simulink model "archSystemMQTT"  (R2021b)
settings: Solver=FixedStepAuto  StartTime=0.0  StopTime=10.0  RelTol=1e-3
settings Model: DataDictionary=theSystem.sldd  Creator=samwarner  LastModifiedBy=samwarner
settings SolverCC: ConcurrentTasks=on

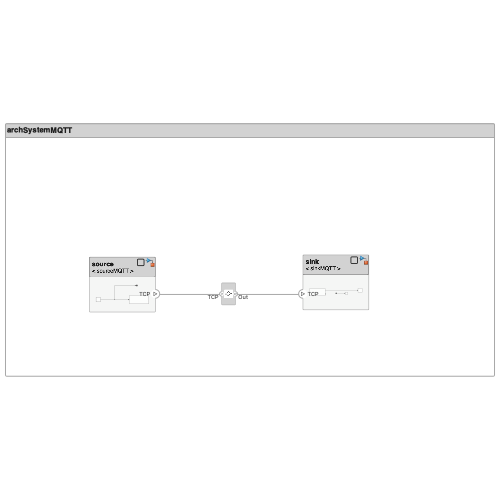
[thumbnail: Simulink's stored preview of the top-level diagram]
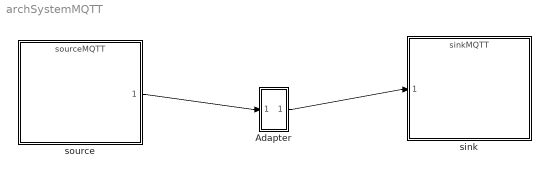
== system archSystemMQTT ==
  Adapter : Subsystem  StartFcn="t  = udpport(\"byte\",'IPV4','LocalHost','0.0.0.0','LocalPort',1090,'EnablePortSharing',true,'ByteOrder', \"little-endian\");"  StopFcn=clear t
      settings: PortSchema="{\"entries\":[{\"content\":{\"margin\":10,\"minimumSpacing\":15,\"sides\":[{\"content\":{\"connectorIds\":[\"In1\"]},\"type\":\"ConnectorPlacement.EquallySpacedRectSide\",\"uuid\":\"7cb3c603-b76a-4abe-bc4c-3d8bbaf6525c\"},{\"content\":{\"connectorIds\":[\"Out1\"],\"side\":\"RIGHT\"},\"type\":\"ConnectorPlacement.EquallySpacedRectSide\",\"uuid\":\"c1f3b5d5-011e-4431-b1e4-f665c8f25138\"},{\"content\":{\"connectorIds\":[],\"side\":\"TOP\"},\"type\":\"ConnectorPlacement.EquallySpacedRectSide\",\"uuid\":\"28d372b1-cf11-4a12-9baa-34993484f63b\"}]},\"type\":\"ConnectorPlacement.EquallySpacedConnector\",\"uuid\":\"e19f808e-9ce7-4910-9971-f476b90c673b\"}],\"packageUris\":[\"http://schema.mathworks.com/mf0/Connector/R2020b\"],\"version\":\"1.0\"}"
  sink : ModelReference  ModelNameDialog=sinkMQTT.slx  SimulationMode=Normal  ModelReferenceVersion=1.11
      settings: PortSchema="{\"entries\":[{\"content\":{\"headerSize\":38,\"margin\":15,\"minimumSpacing\":25,\"sides\":[{\"content\":{\"connectorIds\":[\"In1\"]},\"type\":\"ConnectorPlacement.EquallySpacedRectSide\",\"uuid\":\"a8950277-a1b7-4096-965c-841e51e165a4\"},{\"content\":{\"connectorIds\":[],\"side\":\"RIGHT\"},\"type\":\"ConnectorPlacement.EquallySpacedRectSide\",\"uuid\":\"e2651f39-2f70-4f1f-86f3-2045f7035885\"},{\"content\":{\"connectorIds\":[],\"side\":\"TOP\"},\"type\":\"ConnectorPlacement.EquallySpacedRectSide\",\"uuid\":\"e66f0212-5200-486f-ae88-3f0e7cdde3ab\"}]},\"type\":\"ConnectorPlacement.EquallySpacedConnector\",\"uuid\":\"73cb6547-bcca-43f2-83f0-403e92449084\"}],\"packageUris\":[\"http://schema.mathworks.com/mf0/Connector/R2020b\"],\"version\":\"1.0\"}"
  source : ModelReference  ModelNameDialog=sourceMQTT.slx  SimulationMode=Normal  ModelReferenceVersion=1.11
      settings: PortSchema="{\"entries\":[{\"content\":{\"headerSize\":38,\"margin\":15,\"minimumSpacing\":25,\"sides\":[{\"content\":{\"connectorIds\":[]},\"type\":\"ConnectorPlacement.EquallySpacedRectSide\",\"uuid\":\"a8950277-a1b7-4096-965c-841e51e165a4\"},{\"content\":{\"connectorIds\":[\"Out1\"],\"side\":\"RIGHT\"},\"type\":\"ConnectorPlacement.EquallySpacedRectSide\",\"uuid\":\"e2651f39-2f70-4f1f-86f3-2045f7035885\"},{\"content\":{\"connectorIds\":[],\"side\":\"TOP\"},\"type\":\"ConnectorPlacement.EquallySpacedRectSide\",\"uuid\":\"e66f0212-5200-486f-ae88-3f0e7cdde3ab\"}]},\"type\":\"ConnectorPlacement.EquallySpacedConnector\",\"uuid\":\"73cb6547-bcca-43f2-83f0-403e92449084\"}],\"packageUris\":[\"http://schema.mathworks.com/mf0/Connector/R2020b\"],\"version\":\"1.0\"}"
  wires:
  Adapter/1(Out) -> sink/1
  source/1 -> Adapter/1(TCP)

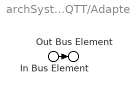
== system archSystemMQTT/Adapter ==
  In Bus Element : Inport  PortName=TCP
  Out Bus Element : Outport  PortName=Out
  wires:
  In Bus Element/1 -> Out Bus Element/1
